simulink model "sampleModel2069_3"  (R2023a)
settings: Solver=VariableStepAuto  StartTime=0.0  StopTime=10.0  RelTol=1e-3
libraries: hdlsllib x4, simulink x2
settings Model: Creator=user1  LastModifiedBy=user1

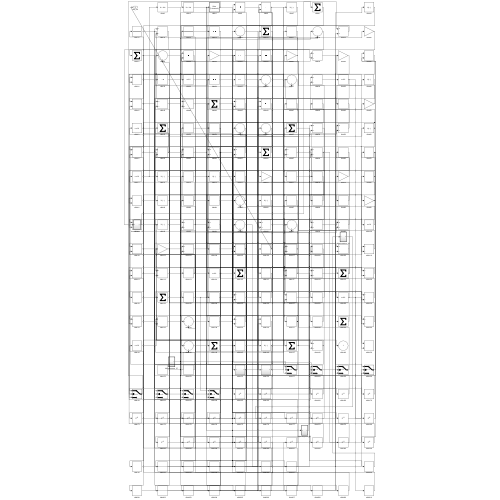
[thumbnail: Simulink's stored preview of the top-level diagram]
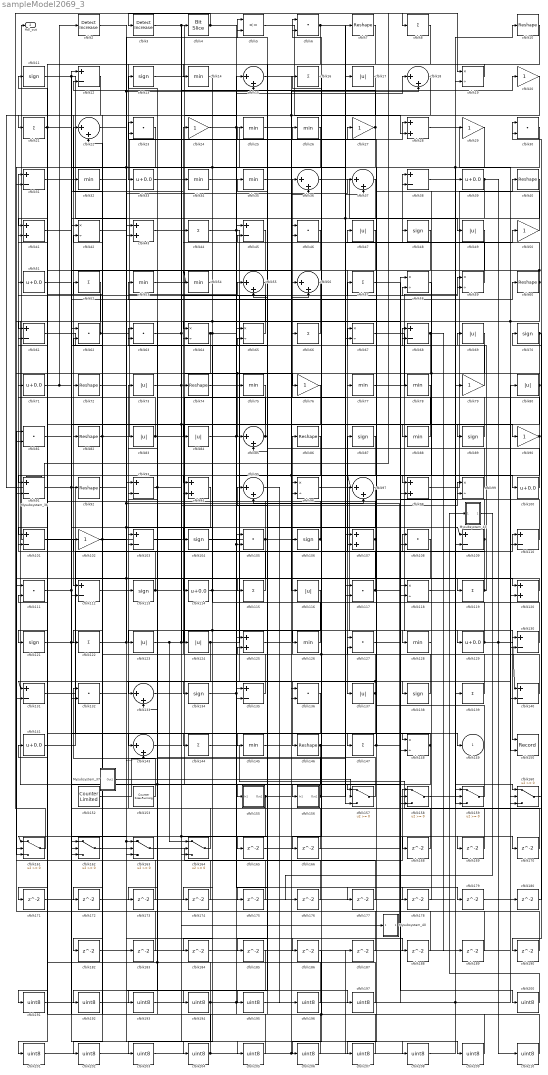
== system sampleModel2069_3 ==
  Mysubsystem_36 : Subsystem  TreatAsAtomicUnit=on  RTWFcnName=Mysubsystem_36
      settings: RTWFcnNameOpts=User specified  RTWFileNameOpts=Use function name
  Mysubsystem_37 : Subsystem  TreatAsAtomicUnit=on  RTWFcnName=Mysubsystem_37
      settings: RTWFcnNameOpts=User specified  RTWFileNameOpts=Use function name
  Mysubsystem_40 : Subsystem  TreatAsAtomicUnit=on  RTWFcnName=Mysubsystem_40
      settings: RTWFcnNameOpts=User specified  RTWFileNameOpts=Use function name
  Mysubsystem_43 : Subsystem  TreatAsAtomicUnit=on  RTWFcnName=Mysubsystem_43
      settings: RTWFcnNameOpts=User specified  RTWFileNameOpts=Use function name
  cfblk{7,10,40,60,72,74,82,86,92,146} (10 alike) : Reshape
  cfblk{33,39,51,71,100,114,129,141} (8 alike) : Bias  Bias=0.0  SaturateOnIntegerOverflow=off
  cfblk{12,31,38,45,61,68,91,93,101,103,109..110,112,130..131,135,140} (17 alike) : Sum  Inputs=+-  OutDataTypeStr=uint8
  cfblk{20,24,27,29,50,76,79,90,102} (9 alike) : Gain  OutDataTypeStr=uint8
  cfblk{11,13,48,70,87,89,104,106,113,121,134,138} (12 alike) : Signum
  cfblk{6,23,30,46,62..63,81,105,108,111,117,127,132,136} (14 alike) : DotProduct  OutDataTypeStr=uint8
  cfblk{28,41,43,94,98,107,120,125} (8 alike) : Sum  OutDataTypeStr=uint8
  cfblk{8,16,21,44,52,57,66,115,119,122,139,144,147} (13 alike) : Sum  Inputs=+  OutDataTypeStr=uint8
  cfblk{17,47,49,69,73,80,83..84,116,123..124,137} (12 alike) : Abs  OutDataTypeStr=uint8  SaturateOnIntegerOverflow=off
  cfblk{19,42,58..59,64..65,67,96,99,118,148} (11 alike) : Product  Inputs=*/  OutDataTypeStr=uint8  RndMeth=Zero  SaturateOnIntegerOverflow=on
  cfblk{14,25..26,32,34..35,53..54,75,77..78,88,126,128,145} (15 alike) : MinMax  OutDataTypeStr=uint8
  cfblk{15,18,22,36..37,55..56,85,95,97,133,143} (12 alike) : Sum  Inputs=|++  OutDataTypeStr=uint8
  cfblk150 : Record  FileSettingsInternal="{\"entries\":[{\"content\":{\"excelSettings\":{\"content\":{},\"type\":\"Streamout.ExcelSettings\"}},\"type\":\"Streamout.FileSettingStorage\",\"uuid\":\"\"}],\"packageUris\":[\"http:\\/\\/schema.mathworks.com\\/mf0\\/streamout_blocks\\/R2020a\"],\"version\":\"1.0\"}"  Layout=[1 1]  SignalsInternal="{\"entries\":[{\"content\":{\"signals\":[{\"content\":{\"blockPath\":[],\"dimensions\":[1],\"domain\":\"\",\"lineColor\":\"#a2142f\",\"plots\":[1],\"port\":1,\"signalID\":61265,\"signalName\":\"cfblk96\"},\"type\":\"RecordBlkView.Signal\",\"uuid\":\"\"},{\"content\":{\"blockPath\":[],\"dimensions\":[1],\"domain\":\"\",\"lineColor\":\"#139fff\",\"plots\":[1],\"port\":2,\"signalID\":61268,\"signalName\":\"cfblk28\"},\"type\":\"RecordBlkView.Signal\",\"uuid\":\"\"}]},\"type\":\"RecordBlkView.InputSignals\",\"uuid\":\"\"}],\"packageUris\":[\"http:\\/\\/schema.mathworks.com\\/mf0\\/streamout_blocks\\/R2020a\"],\"version\":\"1.0\"}"  VisualizationBindings="{\"xyplotplugin\":{\"info\":[{\"series\":[{\"bindingParametersList\":[{\"parameter\":\"X-Axis\",\"signalID\":61265,\"signalName\":\"cfblk96\"},{\"parameter\":\"Y-Axis\",\"signalID\":61268,\"signalName\":\"cfblk28\"}],\"seriesID\":12404}],\"subplotID\":1}]}}"  CompatibilityTag=XY  st=-1
  cfblk152 : hdlsllib/Sources/Counter Limited  uplimit=7  tsamp=-1
  cfblk153 : hdlsllib/Sources/Counter Free-Running  NumBits=16  tsamp=-1
  cfblk155 : Subsystem
      settings: LibrarySourceBlock=|
      | hdlsllib/Ports &
      | Subsystems/Subsystem
  cfblk156 : Subsystem
      settings: LibrarySourceBlock=|
      | hdlsllib/Ports &
      | Subsystems/Subsystem
  cfblk{157..164} (8 alike) : Switch  OutDataTypeStr=uint8  SaturateOnIntegerOverflow=off  InputSameDT=off
  cfblk{165..166,168..180,182..190} (24 alike) : Delay  SampleTime=1
  cfblk{191..197,200..210} (18 alike) : DataTypeConversion  OutDataTypeStr=uint8  SaturateOnIntegerOverflow=off  RndMeth=Floor
  cfblk2 : simulink/Logic and Bit Operations/Detect Increase  vinit=0.0  OutDataTypeStr=uint8
      settings: LibrarySourceBlock=|
      | hdlsllib/Logic and Bit
      | Operations/Detect
      | Increase
  cfblk3 : simulink/Logic and Bit Operations/Detect Increase  vinit=0.0  OutDataTypeStr=uint8
      settings: LibrarySourceBlock=|
      | hdlsllib/Logic and Bit
      | Operations/Detect
      | Increase
  cfblk4 : hdlsllib/Logic and Bit Operations/Bit Slice  lidx=7  ridx=0
  cfblk5 : RelationalOperator  Operator=<=  OutDataTypeStr=boolean  InputSameDT=off
  cfblk149 : Outport  OutDataTypeStr=uint8  VectorParamsAs1DForOutWhenUnconnected=off
  Hdl_out : Outport  Port=2  OutDataTypeStr=uint8
  wires:
  cfblk121/1 -> cfblk149/1, cfblk163/3
  cfblk88/1 -> cfblk36/1
  cfblk12/1 -> cfblk21/1
  cfblk138/1 -> cfblk86/1
  cfblk82/1 -> cfblk28/1, cfblk42/2
  cfblk87/1 -> cfblk137/1
  cfblk52/1 -> cfblk156/1(In1)
  cfblk47/1 -> cfblk127/1
  cfblk146/1 -> cfblk7/1, cfblk162/3
  cfblk48/1 -> cfblk135/2
  cfblk104/1 -> cfblk67/1
  cfblk164/1 -> cfblk73/1
  cfblk126/1 -> cfblk106/1
  cfblk105/1 -> cfblk11/1, cfblk131/2
  cfblk96/1 -> cfblk150/1
  cfblk67/1 -> cfblk129/1
  cfblk117/1 -> cfblk87/1, cfblk130/1
  cfblk98/1 -> cfblk40/1
  cfblk44/1 -> cfblk146/1, cfblk100/1
  cfblk36/1 -> cfblk49/1
  cfblk77/1 -> cfblk59/1
  cfblk124/1 -> cfblk57/1, cfblk133/1
  cfblk161/1 -> cfblk19/1
  cfblk43/1 -> cfblk155/1(In1)
  cfblk3/1 -> Mysubsystem_40/1(In1), cfblk76/1
  cfblk139/1 -> cfblk24/1
  cfblk141/1 -> cfblk108/1
  cfblk66/1 -> cfblk64/1
  cfblk147/1 -> cfblk127/2, cfblk200/1
  cfblk85/1 -> cfblk23/2, cfblk195/1
  cfblk62/1 -> cfblk55/1, cfblk41/2
  cfblk101/1 -> cfblk143/1
  cfblk90/1 -> cfblk35/1, cfblk185/1
  cfblk53/1 -> cfblk116/1
  cfblk158/1 -> cfblk79/1
  cfblk115/1 -> cfblk74/1
  cfblk34/1 -> cfblk128/1
  cfblk83/1 -> cfblk108/2, cfblk71/1
  cfblk37/1 -> cfblk112/1
  cfblk144/1 -> cfblk70/1
  cfblk110/1 -> cfblk47/1
  cfblk17/1 -> cfblk82/1
  cfblk91/1 -> cfblk119/1, cfblk148/1
  cfblk153/1 -> cfblk132/1
  cfblk123/1 -> cfblk17/1, cfblk99/2, cfblk164/1
  cfblk69/1 -> cfblk122/1, cfblk98/1
  cfblk80/1 -> cfblk101/1, cfblk164/2, cfblk77/1
  cfblk8/1 -> cfblk33/1
  cfblk40/1 -> cfblk115/1
  cfblk94/1 -> cfblk112/2
  cfblk59/1 -> cfblk38/1
  cfblk24/1 -> cfblk117/1, cfblk177/1
  cfblk55/1 -> cfblk104/1, cfblk91/2
  cfblk81/1 -> cfblk68/1
  cfblk84/1 -> cfblk139/1, cfblk178/1
  cfblk39/1 -> cfblk67/2, cfblk132/2, cfblk210/1
  cfblk113/1 -> cfblk31/1, cfblk140/2
  cfblk136/1 -> cfblk191/1
  cfblk72/1 -> cfblk93/1
  cfblk22/1 -> cfblk43/1
  cfblk28/1 -> cfblk150/2
  cfblk100/1 -> cfblk63/1
  cfblk50/1 -> cfblk23/1
  cfblk108/1 -> cfblk126/1
  cfblk35/1 -> cfblk97/1, cfblk120/2
  cfblk5/1 -> cfblk28/2
  cfblk26/1 -> cfblk124/1, cfblk161/3
  cfblk75/1 -> cfblk144/1
  cfblk93/1 -> cfblk13/1, cfblk109/2
  cfblk11/1 -> cfblk113/1, cfblk37/2
  cfblk152/1 -> cfblk107/1
  cfblk135/1 -> cfblk103/1
  cfblk112/1 -> cfblk138/1
  cfblk68/1 -> cfblk85/1, cfblk161/2, cfblk189/1
  cfblk33/1 -> cfblk118/1
  cfblk21/1 -> cfblk61/1, cfblk56/2
  cfblk64/1 -> cfblk84/1, cfblk179/1, cfblk171/1
  cfblk119/1 -> cfblk69/1, cfblk101/2
  cfblk54/1 -> cfblk134/1
  cfblk42/1 -> cfblk163/1, cfblk197/1, cfblk117/2
  cfblk155/1(Out1) -> cfblk161/1, cfblk164/3, cfblk110/1
  cfblk63/1 -> cfblk59/2, cfblk120/1
  cfblk13/1 -> cfblk125/1
  cfblk134/1 -> cfblk15/1, cfblk158/2
  cfblk111/1 -> cfblk157/1, cfblk60/1
  cfblk79/1 -> cfblk38/2
  cfblk107/1 -> cfblk25/1, cfblk173/1
  cfblk20/1 -> cfblk72/1
  cfblk60/1 -> cfblk123/1, cfblk110/2, cfblk44/1, cfblk54/1
  cfblk38/1 -> cfblk10/1
  cfblk4/1 -> cfblk3/1, cfblk98/2
  cfblk120/1 -> cfblk114/1
  cfblk159/1 -> cfblk27/1
  cfblk118/1 -> cfblk160/1
  cfblk137/1 -> cfblk52/1, cfblk6/2, cfblk131/1, cfblk157/3
  cfblk14/1 -> cfblk94/1
  cfblk31/1 -> cfblk22/1
  cfblk127/1 -> cfblk99/1
  cfblk73/1 -> cfblk4/1, cfblk130/2
  cfblk163/1 -> cfblk158/1
  cfblk157/1 -> cfblk16/1
  cfblk128/1 -> cfblk48/1
  cfblk130/1 -> cfblk26/1
  cfblk95/1 -> cfblk196/1
  cfblk51/1 -> cfblk34/1
  cfblk7/1 -> cfblk91/1
  cfblk32/1 -> cfblk209/1
  cfblk106/1 -> cfblk94/2, Hdl_out/1
  cfblk103/1 -> cfblk20/1
  cfblk27/1 -> cfblk163/2, cfblk162/2, cfblk12/2
  cfblk49/1 -> cfblk75/1
  cfblk125/1 -> cfblk58/2
  cfblk65/1 -> cfblk51/1
  cfblk2/1 -> cfblk15/2, cfblk143/2
  cfblk140/1 -> cfblk22/2
  cfblk148/1 -> cfblk182/1, cfblk193/1, cfblk145/1
  cfblk114/1 -> cfblk18/1, cfblk184/1
  cfblk25/1 -> cfblk89/1
  cfblk102/1 -> cfblk37/1, cfblk97/2, cfblk109/1, cfblk172/1
  cfblk6/1 -> cfblk43/2, cfblk158/3
  cfblk58/1 -> cfblk88/1
  cfblk99/1 -> cfblk5/1
  cfblk145/1 -> cfblk18/2
  cfblk89/1 -> cfblk6/1
  cfblk109/1 -> cfblk107/2, cfblk53/1
  cfblk15/1 -> cfblk66/1
  cfblk160/1 -> cfblk30/1
  cfblk122/1 -> cfblk5/2, cfblk148/2
  cfblk71/1 -> cfblk90/1, cfblk2/1
  cfblk78/1 -> cfblk194/1
  cfblk56/1 -> cfblk92/1
  cfblk30/1 -> cfblk41/1, cfblk159/3
  cfblk19/1 -> cfblk14/1
  cfblk46/1 -> cfblk201/1
  cfblk23/1 -> cfblk31/2
  cfblk116/1 -> cfblk133/2, cfblk174/1
  cfblk129/1 -> cfblk140/1, cfblk180/1, cfblk64/2
  cfblk156/1(Out1) -> cfblk50/1, cfblk102/1
  cfblk70/1 -> cfblk81/2, cfblk190/1
  cfblk131/1 -> cfblk147/1
  cfblk45/1 -> cfblk204/1
  cfblk18/1 -> Mysubsystem_36/1(In1), cfblk96/2
  cfblk86/1 -> cfblk121/1
  cfblk61/1 -> cfblk65/2
  cfblk10/1 -> cfblk165/1
  cfblk165/1 -> cfblk118/2
  cfblk16/1 -> cfblk166/1
  cfblk166/1 -> cfblk125/2
  cfblk74/1 -> cfblk168/1
  cfblk168/1 -> cfblk135/1
  cfblk57/1 -> cfblk169/1
  cfblk169/1 -> cfblk85/2
  cfblk133/1 -> cfblk170/1
  cfblk170/1 -> cfblk42/1
  cfblk171/1 -> cfblk65/1
  cfblk172/1 -> cfblk159/1
  cfblk173/1 -> cfblk12/1
  cfblk174/1 -> cfblk61/2
  cfblk97/1 -> cfblk175/1
  cfblk175/1 -> cfblk93/2
  cfblk176/1 -> cfblk111/1
  cfblk177/1 -> cfblk55/2
  cfblk178/1 -> cfblk68/2
  cfblk179/1 -> cfblk160/3
  cfblk180/1 -> cfblk30/2
  cfblk182/1 -> cfblk160/2
  cfblk92/1 -> cfblk183/1
  cfblk183/1 -> cfblk81/1
  cfblk184/1 -> cfblk36/2
  cfblk162/1 -> cfblk186/1
  cfblk187/1 -> cfblk62/2
  cfblk132/1 -> cfblk188/1
  cfblk188/1 -> cfblk58/1
  cfblk189/1 -> cfblk103/2
  cfblk190/1 -> cfblk159/2
  cfblk191/1 -> cfblk80/1, cfblk39/1, cfblk105/2, cfblk105/1
  cfblk185/1 -> cfblk192/1
  cfblk192/1 -> cfblk136/1
  cfblk193/1 -> cfblk136/2
  cfblk194/1 -> cfblk111/2, cfblk203/1
  cfblk195/1 -> cfblk78/1
  cfblk196/1 -> cfblk63/2, cfblk62/1
  cfblk197/1 -> cfblk95/1
  cfblk201/1 -> cfblk19/2, cfblk96/1
  cfblk76/1 -> cfblk202/1
  cfblk202/1 -> cfblk46/1
  cfblk203/1 -> cfblk46/2
  cfblk204/1 -> cfblk187/1, cfblk162/1
  cfblk143/1 -> cfblk205/1
  cfblk205/1 -> cfblk45/1
  cfblk186/1 -> cfblk206/1
  cfblk206/1 -> cfblk45/2
  cfblk29/1 -> cfblk207/1
  cfblk207/1 -> cfblk141/1
  cfblk41/1 -> cfblk208/1
  cfblk208/1 -> cfblk29/1
  cfblk209/1 -> cfblk83/1, cfblk56/1
  cfblk210/1 -> cfblk32/1
  Mysubsystem_36/1(y) -> cfblk8/1
  Mysubsystem_37/1(Out1) -> cfblk157/2
  Mysubsystem_40/1(Out1) -> cfblk95/2
  cfblk200/1 -> Mysubsystem_43/1(In1)
  Mysubsystem_43/1(Out1) -> cfblk176/1

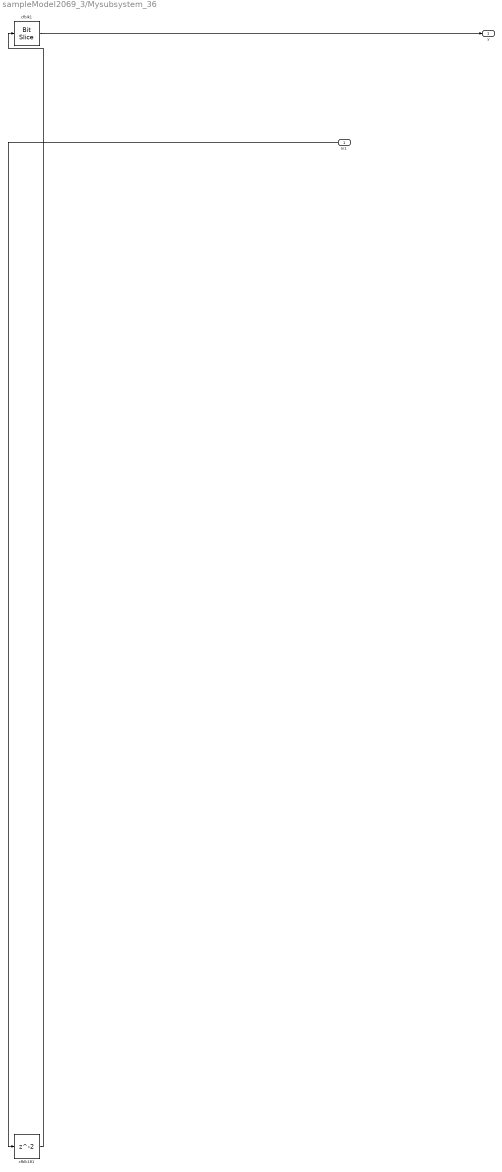
== system sampleModel2069_3/Mysubsystem_36 ==
  In1 : Inport
  cfblk1 : hdlsllib/Logic and Bit Operations/Bit Slice  lidx=7  ridx=0
  cfblk181 : Delay  SampleTime=1
  y : Outport
  wires:
  In1/1 -> cfblk181/1
  cfblk181/1 -> cfblk1/1
  cfblk1/1 -> y/1

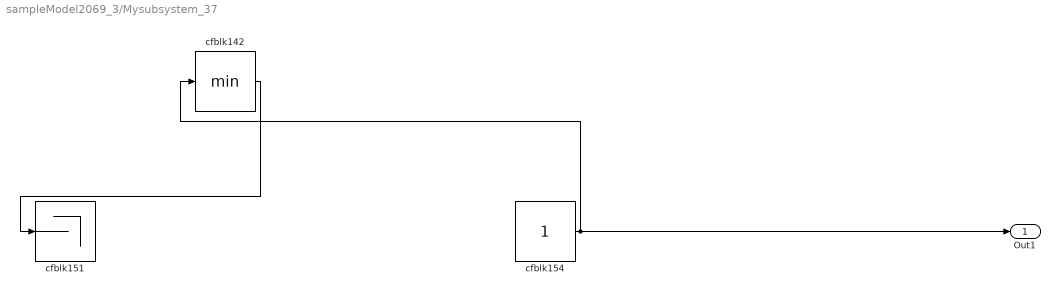
== system sampleModel2069_3/Mysubsystem_37 ==
  cfblk142 : MinMax
  cfblk151 : Terminator
  cfblk154 : Constant  SampleTime=-1
  Out1 : Outport
  wires:
  cfblk142/1 -> cfblk151/1
  cfblk154/1 -> Out1/1, cfblk142/1

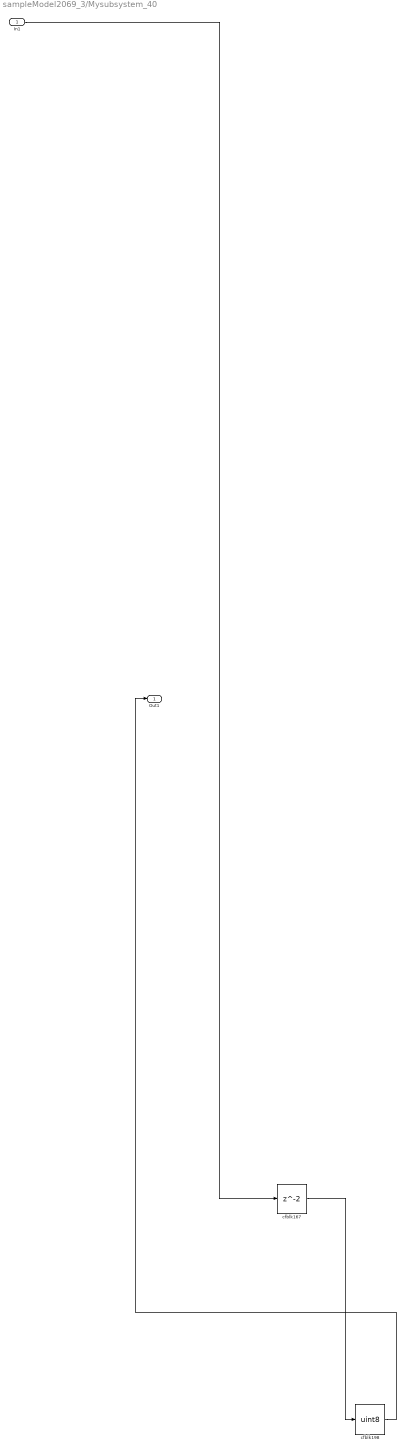
== system sampleModel2069_3/Mysubsystem_40 ==
  In1 : Inport
  cfblk167 : Delay  SampleTime=1
  cfblk198 : DataTypeConversion  OutDataTypeStr=uint8  SaturateOnIntegerOverflow=off  RndMeth=Floor
  Out1 : Outport
  wires:
  cfblk198/1 -> Out1/1
  cfblk167/1 -> cfblk198/1
  In1/1 -> cfblk167/1

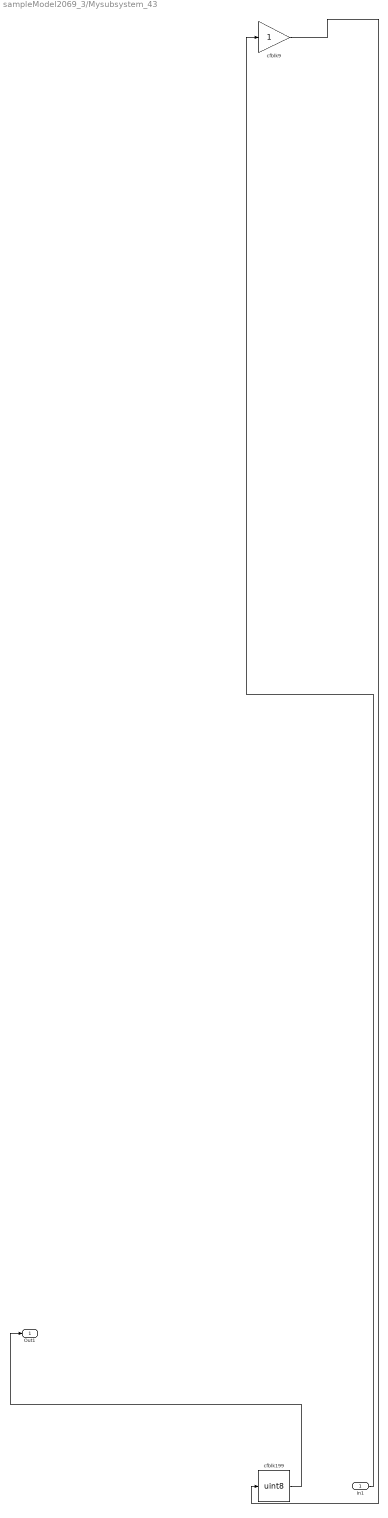
== system sampleModel2069_3/Mysubsystem_43 ==
  In1 : Inport
  cfblk199 : DataTypeConversion  OutDataTypeStr=uint8  SaturateOnIntegerOverflow=off  RndMeth=Floor
  cfblk9 : Gain
  Out1 : Outport
  wires:
  cfblk9/1 -> cfblk199/1
  In1/1 -> cfblk9/1
  cfblk199/1 -> Out1/1

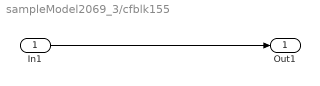
== system sampleModel2069_3/cfblk155 ==
  In1 : Inport
  Out1 : Outport
  wires:
  In1/1 -> Out1/1

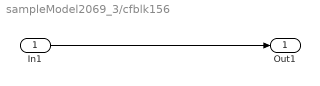
== system sampleModel2069_3/cfblk156 ==
  In1 : Inport
  Out1 : Outport
  wires:
  In1/1 -> Out1/1
